simulink model "ThreeFazAlgorythmNew"  (Simulink 8.3)
settings: Solver=ode4  StartTime=0.0  StopTime=2  FixedStep=0.0001  RelTol=1e-3
settings Model: Creator=Admin  LastModifiedBy=Engine
settings DataIOCC: SignalLoggingSaveFormat=Dataset
settings OptimizationCC: ExpressionDepthLimit=2147483647
settings DebuggingCC: SaveWithParameterizedLinksMsg=none  FcnCallInpInsideContextMsg=UseLocalSettings
settings SFSimCC: SimParseCustomCode=off
settings RTWCC: IncludeERTFirstTime=on

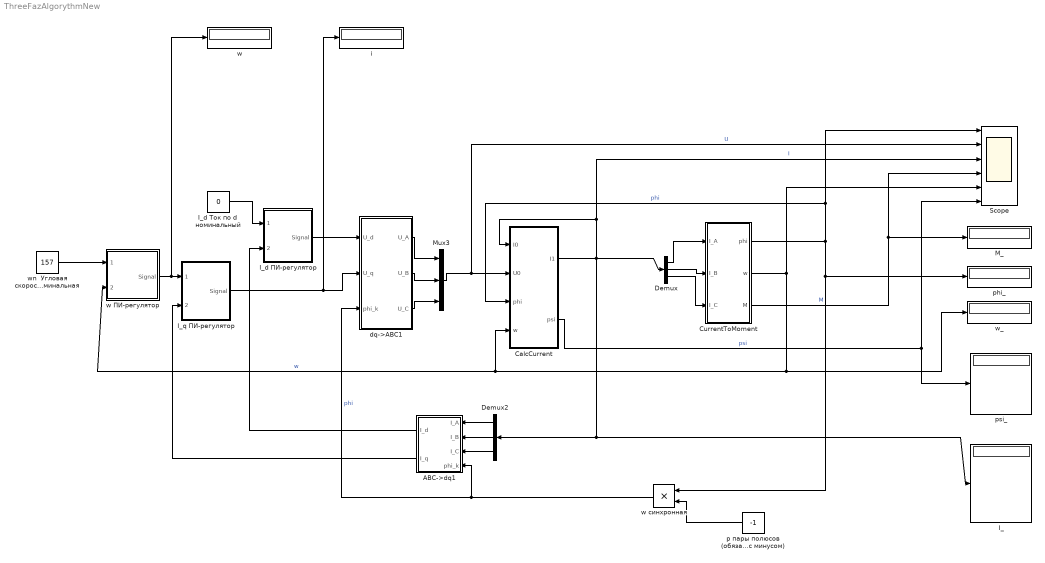
== system ThreeFazAlgorythmNew ==
  " I_d ПИ-регулятор " : Subsystem  mask{K=0.298*0.05, Limit=100000000, T=2.495*0.05}
  ABC->dq1 : Subsystem
  CalcCurrent : Subsystem  mask{Rs=0.0152*2, CoerPower=860000, VitkiNum=63, I_n=29, FazCount=3}
  CurrentToMoment : Subsystem  mask{J=0.007137, w0=50, Mc=24*0+5, Phi0=(115)*pi/180}
  Demux : Demux  Outputs=3
  Demux2 : Demux  Outputs=3
  I_ : Display
  I_d Ток по d  номинальный : Constant  Value=0
  "I_q ПИ-регулятор " : Subsystem  mask{K=0.298*0.05, Limit=10000000, T=2.495*0.05}
  M_ : Display
  Mux3 : Mux  Inputs=3
  Scope : Scope  NumInputPorts=6
      settings: TimeRange=0.3  YMin=2.5~-25~-150~-0.15~-100~-0.15  YMax=22.5~25~150~0.025~400~0.15
  dq->ABC1 : Subsystem
  i : Display
  p пары полюсов (обязательно c минусом) : Constant  Value=-1
  phi_ : Display
  psi_ : Display
  w : Display
  w ПИ-регулятор : Subsystem  mask{K=22.764*0.05, Limit=500, T=1897*0.05}
  w синхронная : Product  RndMeth=Zero
  w_ : Display
  wn  Угловая скорость  номинальная : Constant  Value=157
  wires:
  wn  Угловая скорость  номинальная/1 -> w ПИ-регулятор/1(Nominal)
  I_d Ток по d  номинальный/1 -> " I_d ПИ-регулятор "/1(Nominal)
  w ПИ-регулятор/1(Signal) -> w/1, "I_q ПИ-регулятор "/1(Nominal)
  " I_d ПИ-регулятор "/1(Signal) -> dq->ABC1/1(U_d)
  "I_q ПИ-регулятор "/1(Signal) -> dq->ABC1/2(U_q), i/1
  dq->ABC1/1(U_A) -> Mux3/1
  dq->ABC1/2(U_B) -> Mux3/2
  dq->ABC1/3(U_C) -> Mux3/3
  Mux3/1 -> Scope/2, CalcCurrent/2(U0)  "U"
  Demux/1 -> CurrentToMoment/1(I_A)
  Demux/2 -> CurrentToMoment/2(I_B)
  Demux/3 -> CurrentToMoment/3(I_C)
  CalcCurrent/2(psi) -> psi_/1, Scope/6  "psi"
  CurrentToMoment/3(M) -> Scope/4, M_/1  "M"
  CalcCurrent/1(I1) -> I_/1, Demux2/1, Demux/1, Scope/3, CalcCurrent/1(I0)  "I"
  Demux2/1 -> ABC->dq1/1(I_A)
  Demux2/2 -> ABC->dq1/2(I_B)
  Demux2/3 -> ABC->dq1/3(I_C)
  CurrentToMoment/2(w) -> w ПИ-регулятор/2(Current), CalcCurrent/4(w), w_/1, Scope/5  "w"
  CurrentToMoment/1(phi) -> Scope/1, CalcCurrent/3(phi), w синхронная/1, phi_/1  "phi"
  p пары полюсов (обязательно c минусом)/1 -> w синхронная/2
  w синхронная/1 -> dq->ABC1/3(phi_k), ABC->dq1/4(phi_k)  "phi"
  ABC->dq1/2(I_q) -> "I_q ПИ-регулятор "/2(Current)
  ABC->dq1/1(I_d) -> " I_d ПИ-регулятор "/2(Current)

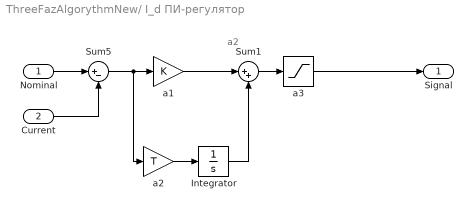
== system ThreeFazAlgorythmNew/ I_d ПИ-регулятор  ==
  note: a2
  Nominal : Inport
  Current : Inport  Port=2
  Integrator : Integrator  LimitOutput=on  UpperSaturationLimit=Limit  LowerSaturationLimit=-Limit
  Sum1 : Sum  Inputs=|++
  Sum5 : Sum  Inputs=|+-
  a1 : Gain  Gain=K
  a2 : Gain  Gain=T
  a3 : Saturate  UpperLimit=Limit  LowerLimit=-Limit
  Signal : Outport
  wires:
  a1/1 -> Sum1/1
  a2/1 -> Integrator/1
  Integrator/1 -> Sum1/2
  Sum1/1 -> a3/1
  a3/1 -> Signal/1
  Sum5/1 -> a2/1, a1/1
  Nominal/1 -> Sum5/1
  Current/1 -> Sum5/2

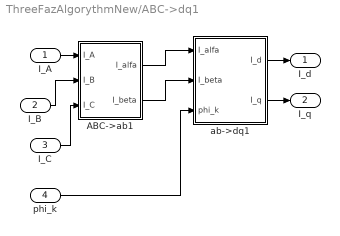
== system ThreeFazAlgorythmNew/ABC->dq1 ==
  I_A : Inport
  I_B : Inport  Port=2
  I_C : Inport  Port=3
  phi_k : Inport  Port=4
  ABC->ab1 : Subsystem
  ab->dq1 : Subsystem
  I_d : Outport
  I_q : Outport  Port=2
  wires:
  ABC->ab1/1(I_alfa) -> ab->dq1/1(I_alfa)
  ABC->ab1/2(I_beta) -> ab->dq1/2(I_beta)
  I_A/1 -> ABC->ab1/1(I_A)
  ab->dq1/1(I_d) -> I_d/1
  I_B/1 -> ABC->ab1/2(I_B)
  ab->dq1/2(I_q) -> I_q/1
  I_C/1 -> ABC->ab1/3(I_C)
  phi_k/1 -> ab->dq1/3(phi_k)

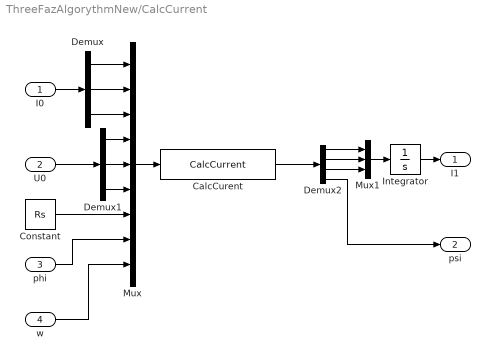
== system ThreeFazAlgorythmNew/CalcCurrent ==
  I0 : Inport
  U0 : Inport  Port=2
  phi : Inport  Port=3
  w : Inport  Port=4
  CalcCurent : S-Function  FunctionName=CalcCurrent  Parameters=CoerPower, VitkiNum, I_n, FazCount  EnableBusSupport=off
  Constant : Constant  Value=Rs
  Demux : Demux  Outputs=3
  Demux1 : Demux  Outputs=3
  Demux2 : Demux
  Integrator : Integrator
  Mux : Mux  Inputs=9
  Mux1 : Mux  Inputs=3
  I1 : Outport
  psi : Outport  Port=2
  wires:
  Mux/1 -> CalcCurent/1
  Demux/2 -> Mux/2
  Demux/1 -> Mux/1
  Demux/3 -> Mux/3
  I0/1 -> Demux/1
  Demux1/2 -> Mux/5
  Demux1/1 -> Mux/4
  Demux1/3 -> Mux/6
  U0/1 -> Demux1/1
  phi/1 -> Mux/8
  Constant/1 -> Mux/7
  w/1 -> Mux/9
  CalcCurent/1 -> Demux2/1
  Demux2/1 -> Mux1/1
  Demux2/2 -> Mux1/2
  Demux2/3 -> Mux1/3
  Demux2/4 -> psi/1
  Mux1/1 -> Integrator/1
  Integrator/1 -> I1/1

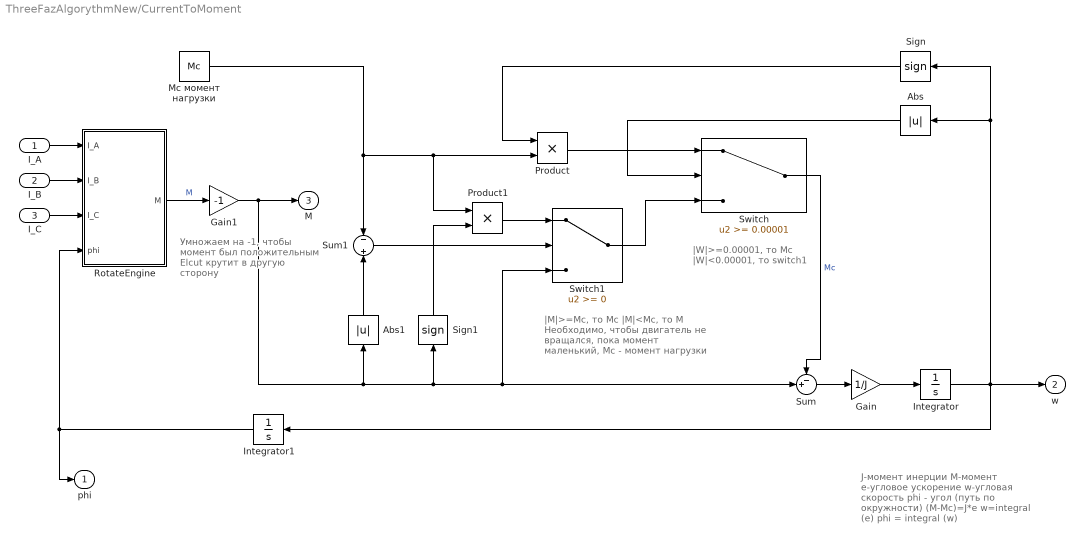
== system ThreeFazAlgorythmNew/CurrentToMoment ==
  note: Умножаем на -1,
      | чтобы момент
      | был положительным
      | Elcut крутит в
      | другую сторону
  note: J-момент инерции
      | M-момент
      | e-угловое ускорение
      | w-угловая скорость
      | phi - угол (путь по окружности)
      |
      | (M-Mc)=J*e
      | w=integral (e)
      | phi = integral (w)
  note: |W|>=0.00001, то Mc
      | |W|<0.00001, то switch1
  note: |M|>=Mс, то Mс
      | |M|<Mс, то M
      | Необходимо, чтобы двигатель
      | не вращался, пока
      | момент маленький,
      | Mc - момент нагрузки
  I_A : Inport
  I_B : Inport  Port=2
  I_C : Inport  Port=3
  Abs : Abs
  Abs1 : Abs
  Gain : Gain  Gain=1/J
  Gain1 : Gain  Gain=-1
  Integrator : Integrator  InitialCondition=w0
  Integrator1 : Integrator  InitialCondition=Phi0
  Mс момент нагрузки : Constant  Value=Mc
  Product : Product  RndMeth=Zero
  Product1 : Product  RndMeth=Zero
  RotateEngine : Subsystem
  Sign : Signum
  Sign1 : Signum
  Sum : Sum  Inputs=-+|
  Sum1 : Sum  Inputs=-||+
  Switch : Switch  Threshold=0.00001
  Switch1 : Switch
  phi : Outport
  w : Outport  Port=2
  M : Outport  Port=3
  wires:
  I_A/1 -> RotateEngine/1(I_A)
  I_B/1 -> RotateEngine/2(I_B)
  I_C/1 -> RotateEngine/3(I_C)
  Integrator1/1 -> RotateEngine/4(phi), phi/1
  RotateEngine/1(M) -> Gain1/1  "M"
  Switch1/1 -> Switch/3
  Product/1 -> Switch/1
  Mс момент нагрузки/1 -> Sum1/1, Product/2, Product1/1
  Switch/1 -> Sum/1  "Mс"
  Sum/1 -> Gain/1
  Gain/1 -> Integrator/1
  Integrator/1 -> Abs/1, Sign/1, w/1, Integrator1/1
  Abs/1 -> Switch/2
  Sign/1 -> Product/1
  Abs1/1 -> Sum1/2
  Sum1/1 -> Switch1/2
  Product1/1 -> Switch1/1
  Sign1/1 -> Product1/2
  Gain1/1 -> Abs1/1, Sum/2, Switch1/3, Sign1/1, M/1

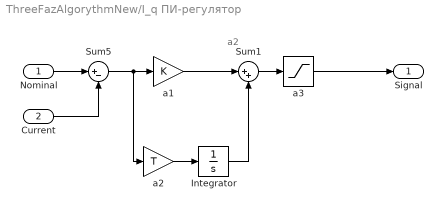
== system ThreeFazAlgorythmNew/I_q ПИ-регулятор  ==
  note: a2
  Nominal : Inport
  Current : Inport  Port=2
  Integrator : Integrator  LimitOutput=on  UpperSaturationLimit=Limit  LowerSaturationLimit=-Limit
  Sum1 : Sum  Inputs=|++
  Sum5 : Sum  Inputs=|+-
  a1 : Gain  Gain=K
  a2 : Gain  Gain=T
  a3 : Saturate  UpperLimit=Limit  LowerLimit=-Limit
  Signal : Outport
  wires:
  Current/1 -> Sum5/2
  Nominal/1 -> Sum5/1
  Sum5/1 -> a1/1, a2/1
  a3/1 -> Signal/1
  Sum1/1 -> a3/1
  Integrator/1 -> Sum1/2
  a2/1 -> Integrator/1
  a1/1 -> Sum1/1

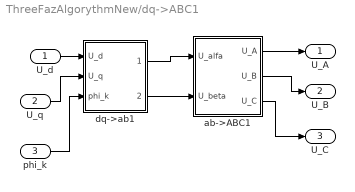
== system ThreeFazAlgorythmNew/dq->ABC1 ==
  U_d : Inport
  U_q : Inport  Port=2
  phi_k : Inport  Port=3
  ab->ABC1 : Subsystem
  dq->ab1 : Subsystem
  U_A : Outport
  U_B : Outport  Port=2
  U_C : Outport  Port=3
  wires:
  ab->ABC1/3(U_C) -> U_C/1
  phi_k/1 -> dq->ab1/3(phi_k)
  ab->ABC1/2(U_B) -> U_B/1
  U_q/1 -> dq->ab1/2(U_q)
  U_d/1 -> dq->ab1/1(U_d)
  ab->ABC1/1(U_A) -> U_A/1
  dq->ab1/2(U_beta) -> ab->ABC1/2(U_beta)
  dq->ab1/1(U_alfa) -> ab->ABC1/1(U_alfa)

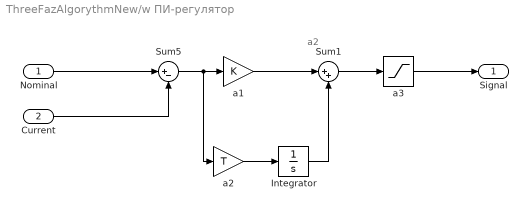
== system ThreeFazAlgorythmNew/w ПИ-регулятор ==
  note: a2
  Nominal : Inport
  Current : Inport  Port=2
  Integrator : Integrator  LimitOutput=on  UpperSaturationLimit=Limit  LowerSaturationLimit=-Limit
  Sum1 : Sum  Inputs=|++
  Sum5 : Sum  Inputs=|+-
  a1 : Gain  Gain=K
  a2 : Gain  Gain=T
  a3 : Saturate  UpperLimit=Limit  LowerLimit=-Limit
  Signal : Outport
  wires:
  Nominal/1 -> Sum5/1
  Sum5/1 -> a1/1, a2/1
  a3/1 -> Signal/1
  Sum1/1 -> a3/1
  Integrator/1 -> Sum1/2
  a2/1 -> Integrator/1
  a1/1 -> Sum1/1
  Current/1 -> Sum5/2

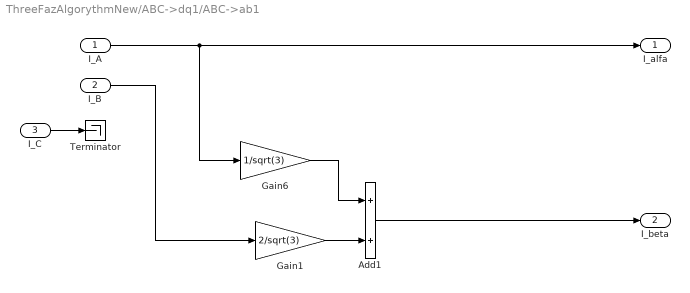
== system ThreeFazAlgorythmNew/ABC->dq1/ABC->ab1 ==
  I_A : Inport
  I_B : Inport  Port=2
  I_C : Inport  Port=3
  Add1 : Sum
  Gain1 : Gain  Gain=2/sqrt(3)
  Gain6 : Gain  Gain=1/sqrt(3)
  Terminator : Terminator
  I_alfa : Outport
  I_beta : Outport  Port=2
  wires:
  I_A/1 -> Gain6/1, I_alfa/1
  Add1/1 -> I_beta/1
  Gain6/1 -> Add1/1
  Gain1/1 -> Add1/2
  I_B/1 -> Gain1/1
  I_C/1 -> Terminator/1

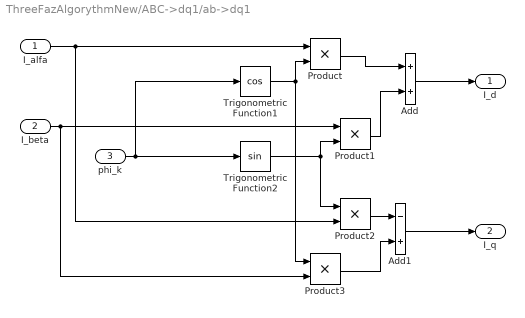
== system ThreeFazAlgorythmNew/ABC->dq1/ab->dq1 ==
  I_alfa : Inport
  I_beta : Inport  Port=2
  phi_k : Inport  Port=3
  Add : Sum
  Add1 : Sum  Inputs=-+
  Product{,1..3} (4 alike) : Product  RndMeth=Zero
  Trigonometric Function1 : Trigonometry  Operator=cos
  Trigonometric Function2 : Trigonometry
  I_d : Outport
  I_q : Outport  Port=2
  wires:
  Add1/1 -> I_q/1
  Product3/1 -> Add1/2
  Product1/1 -> Add/2
  Product2/1 -> Add1/1
  Add/1 -> I_d/1
  Product/1 -> Add/1
  I_beta/1 -> Product3/2, Product1/1
  Trigonometric Function2/1 -> Product2/1, Product1/2
  phi_k/1 -> Trigonometric Function2/1, Trigonometric Function1/1
  Trigonometric Function1/1 -> Product3/1, Product/2
  I_alfa/1 -> Product2/2, Product/1

== system ThreeFazAlgorythmNew/CurrentToMoment/RotateEngine ==
  I_A : Inport
  I_B : Inport  Port=2
  I_C : Inport  Port=3
  phi : Inport  Port=4
  S-Function : S-Function  FunctionName=RotateEngineInElcut  EnableBusSupport=off
  Vector Concatenate : Concatenate  NumInputs=4
  M : Outport
  wires:
  Vector Concatenate/1 -> S-Function/1
  I_A/1 -> Vector Concatenate/1
  S-Function/1 -> M/1
  I_B/1 -> Vector Concatenate/2
  I_C/1 -> Vector Concatenate/3
  phi/1 -> Vector Concatenate/4

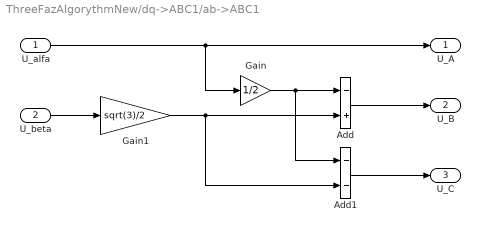
== system ThreeFazAlgorythmNew/dq->ABC1/ab->ABC1 ==
  U_alfa : Inport
  U_beta : Inport  Port=2
  Add : Sum  Inputs=-+
  Add1 : Sum  Inputs=--
  Gain : Gain  Gain=1/2
  Gain1 : Gain  Gain=sqrt(3)/2
  U_A : Outport
  U_B : Outport  Port=2
  U_C : Outport  Port=3
  wires:
  Add1/1 -> U_C/1
  Add/1 -> U_B/1
  U_alfa/1 -> U_A/1, Gain/1
  U_beta/1 -> Gain1/1
  Gain/1 -> Add/1, Add1/1
  Gain1/1 -> Add/2, Add1/2

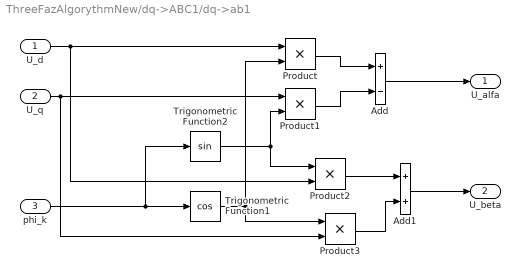
== system ThreeFazAlgorythmNew/dq->ABC1/dq->ab1 ==
  U_d : Inport
  U_q : Inport  Port=2
  phi_k : Inport  Port=3
  Add : Sum  Inputs=+-
  Add1 : Sum
  Product{,1..3} (4 alike) : Product  RndMeth=Zero
  Trigonometric Function1 : Trigonometry  Operator=cos
  Trigonometric Function2 : Trigonometry
  U_alfa : Outport
  U_beta : Outport  Port=2
  wires:
  Add1/1 -> U_beta/1
  Product3/1 -> Add1/2
  Product2/1 -> Add1/1
  Add/1 -> U_alfa/1
  Product1/1 -> Add/2
  Product/1 -> Add/1
  U_q/1 -> Product3/2, Product1/1
  Trigonometric Function2/1 -> Product2/1, Product1/2
  U_d/1 -> Product2/2, Product/1
  Trigonometric Function1/1 -> Product3/1, Product/2
  phi_k/1 -> Trigonometric Function1/1, Trigonometric Function2/1
